simulink model "Robust_design_step_validation_2_2_4"  (R2024b)
settings: Solver=VariableStepAuto  StartTime=0.0  StopTime=20  FixedStep=0.001  RelTol=1e-3
undefined symbols (not defined in the file): degs2rpm, drv, gbox, index, K_vec, mld, mot, Nu, Nx, rads2rpm, rdp, rpm2rads, sens, Ts, u_bar_max
settings Model: Creator=Enrico  LastModifiedBy=Enrico 2
settings DataIOCC: ReturnWorkspaceOutputsName=out_black_box

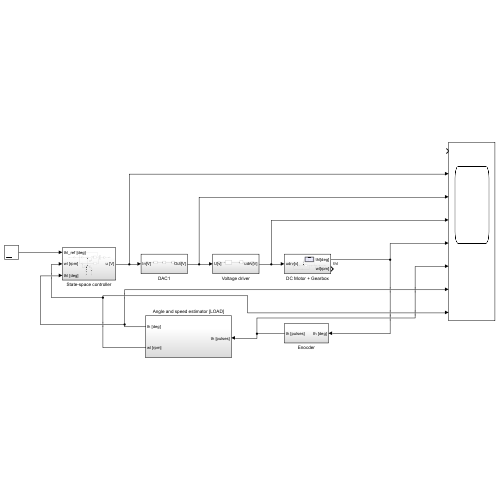
[thumbnail: Simulink's stored preview of the top-level diagram]
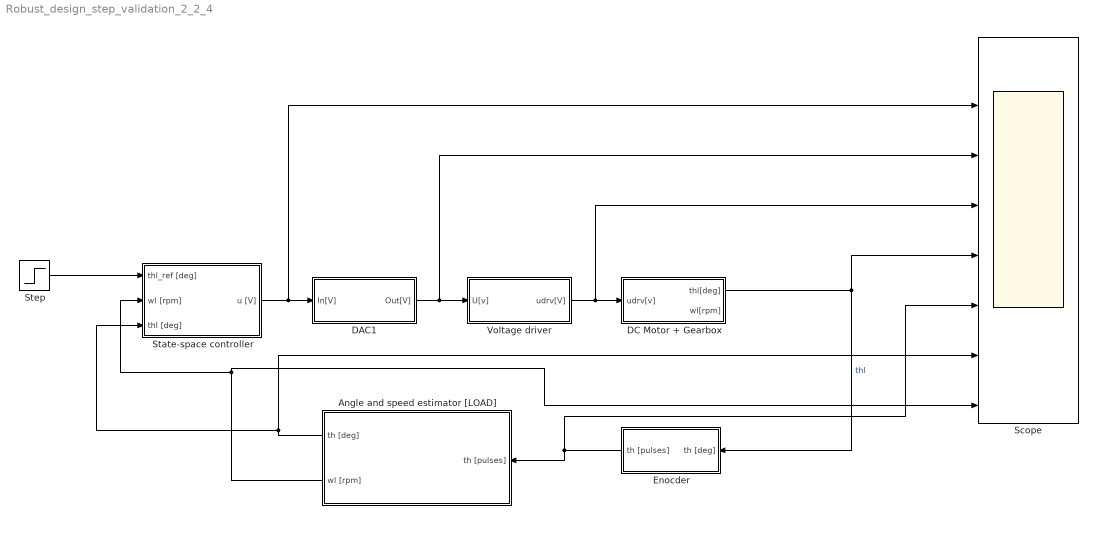
== system Robust_design_step_validation_2_2_4 ==
  Angle and speed estimator [LOAD] : Subsystem
  DAC1 : Subsystem
  DC Motor + Gearbox : Subsystem
  Enocder : Subsystem
  Scope : Scope  NumInputPorts=8
  State-space controller : Subsystem
  Step : Step  After=120  SampleTime=0
  Voltage driver : Subsystem
  wires:
  State-space controller/1(u [V]) -> DAC1/1(In[V]), Scope/2
  DAC1/1(Out[V]) -> Voltage driver/1(U[v]), Scope/3
  Step/1 -> State-space controller/1(thl_ref [deg])
  Enocder/1(th [pulses]) -> Scope/6, Angle and speed estimator [LOAD]/1(th [pulses])
  Voltage driver/1(udrv[V]) -> DC Motor + Gearbox/1(udrv[v]), Scope/4
  Angle and speed estimator [LOAD]/1(th [deg]) -> Scope/7, State-space controller/3(thl [deg])
  Angle and speed estimator [LOAD]/2(wl [rpm]) -> State-space controller/2(wl [rpm]), Scope/8
  DC Motor + Gearbox/1(thl[deg]) -> Enocder/1(th [deg]), Scope/5  "thl"

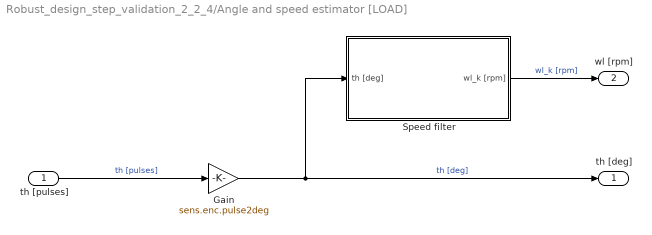
== system Robust_design_step_validation_2_2_4/Angle and speed estimator [LOAD] ==
  th [pulses] : Inport
  Gain : Gain  Gain=sens.enc.pulse2deg
  Speed filter : Subsystem
  th [deg] : Outport
  wl [rpm] : Outport  Port=2
  wires:
  Speed filter/1(wl_k [rpm]) -> wl [rpm]/1  "wl_k [rpm]"
  th [pulses]/1 -> Gain/1  "th [pulses]"
  Gain/1 -> Speed filter/1(th [deg]), th [deg]/1  "th [deg]"

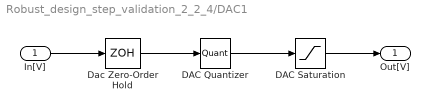
== system Robust_design_step_validation_2_2_4/DAC1 ==
  In[V] : Inport
  DAC Quantizer : Quantizer  QuantizationInterval=20/(2^16-1)
  DAC Saturation : Saturate  UpperLimit=10  LowerLimit=-10
  Dac Zero-Order Hold : ZeroOrderHold  SampleTime=Ts
  Out[V] : Outport
  wires:
  In[V]/1 -> Dac Zero-Order Hold/1
  DAC Saturation/1 -> Out[V]/1
  DAC Quantizer/1 -> DAC Saturation/1
  Dac Zero-Order Hold/1 -> DAC Quantizer/1

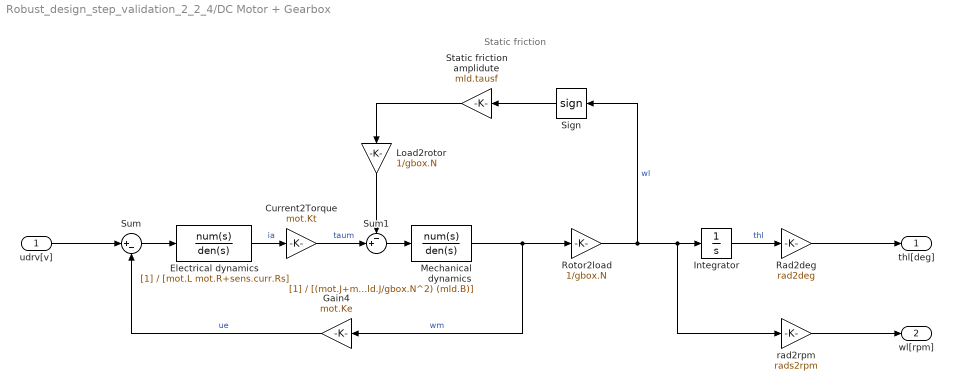
== system Robust_design_step_validation_2_2_4/DC Motor + Gearbox ==
  note: Static friction
  udrv[v] : Inport
  " Sign" : Signum  ZeroCross=off
  Current2Torque : Gain  Gain=mot.Kt
  Electrical dynamics : TransferFcn  Denominator=[mot.L mot.R+sens.curr.Rs]
  Gain4 : Gain  Gain=mot.Ke
  Integrator : Integrator
  Load2rotor : Gain  Gain=1/gbox.N
  Mechanical dynamics : TransferFcn  Denominator=[(mot.J+mld.J/gbox.N^2) (mld.B)]
  Rad2deg : Gain  Gain=rad2deg
  Rotor2load : Gain  Gain=1/gbox.N
  Static friction amplidute : Gain  Gain=mld.tausf
  Sum : Sum  Inputs=|+-
  Sum1 : Sum  Inputs=-+|
  rad2rpm : Gain  Gain=rads2rpm
  thl[deg] : Outport
  wl[rpm] : Outport  Port=2
  wires:
  udrv[v]/1 -> Sum/1
  Sum/1 -> Electrical dynamics/1
  Electrical dynamics/1 -> Current2Torque/1  "ia"
  Current2Torque/1 -> Sum1/2  "taum"
  Load2rotor/1 -> Sum1/1
  " Sign"/1 -> Static friction amplidute/1
  Static friction amplidute/1 -> Load2rotor/1
  Sum1/1 -> Mechanical dynamics/1
  Mechanical dynamics/1 -> Gain4/1, Rotor2load/1  "wm"
  Gain4/1 -> Sum/2  "ue"
  Rad2deg/1 -> thl[deg]/1
  rad2rpm/1 -> wl[rpm]/1
  Integrator/1 -> Rad2deg/1  "thl"
  Rotor2load/1 -> " Sign"/1, rad2rpm/1, Integrator/1  "wl"

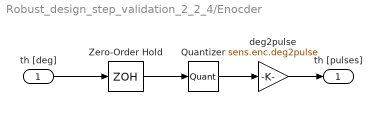
== system Robust_design_step_validation_2_2_4/Enocder ==
  th [deg] : Inport
  Quantizer : Quantizer  QuantizationInterval=sens.enc.pulse2deg
  Zero-Order Hold : ZeroOrderHold  SampleTime=Ts
  deg2pulse : Gain  Gain=sens.enc.deg2pulse
  th [pulses] : Outport
  wires:
  Quantizer/1 -> deg2pulse/1
  th [deg]/1 -> Zero-Order Hold/1
  Zero-Order Hold/1 -> Quantizer/1
  deg2pulse/1 -> th [pulses]/1

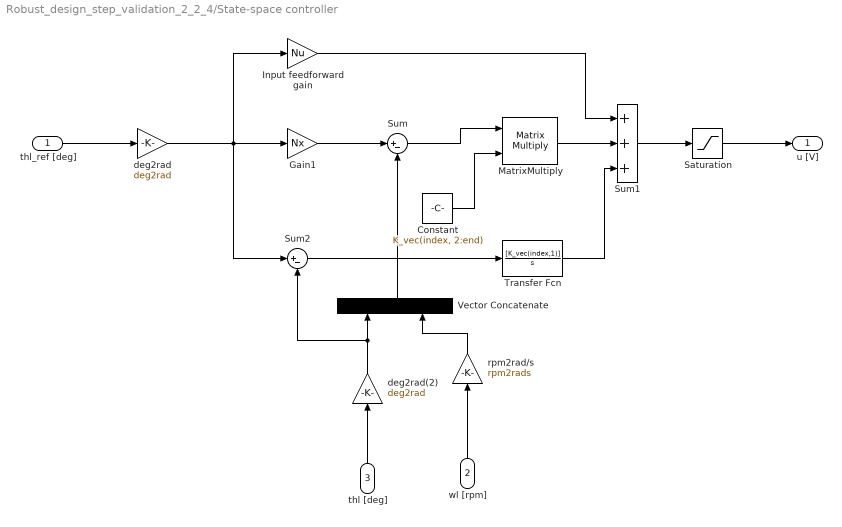
== system Robust_design_step_validation_2_2_4/State-space controller ==
  thl_ref [deg] : Inport
  wl [rpm] : Inport  Port=2
  thl [deg] : Inport  Port=3
  Constant : Constant  Value=K_vec(index, 2:end)
  Gain1 : Gain  Gain=Nx
  Input feedforward gain : Gain  Gain=Nu
  MatrixMultiply : Product  Multiplication=Matrix(*)
  Saturation : Saturate  UpperLimit=u_bar_max  LowerLimit=-u_bar_max
  Sum : Sum  Inputs=|+-
  Sum1 : Sum  Inputs=+++
  Sum2 : Sum  Inputs=|+-
  Transfer Fcn : TransferFcn  Numerator=[K_vec(index,1)]  Denominator=[1 0]
  Vector Concatenate : Concatenate
  deg2rad : Gain  Gain=deg2rad
  deg2rad(2) : Gain  Gain=deg2rad
  rpm2rad/s : Gain  Gain=rpm2rads
  u [V] : Outport
  wires:
  Gain1/1 -> Sum/1
  Sum1/1 -> Saturation/1
  deg2rad/1 -> Gain1/1, Sum2/1, Input feedforward gain/1
  thl_ref [deg]/1 -> deg2rad/1
  wl [rpm]/1 -> rpm2rad/s/1
  Input feedforward gain/1 -> Sum1/1
  Vector Concatenate/1 -> Sum/2
  Saturation/1 -> u [V]/1
  Sum/1 -> MatrixMultiply/1
  Constant/1 -> MatrixMultiply/2
  MatrixMultiply/1 -> Sum1/2
  Transfer Fcn/1 -> Sum1/3
  Sum2/1 -> Transfer Fcn/1
  thl [deg]/1 -> deg2rad(2)/1
  deg2rad(2)/1 -> Vector Concatenate/1, Sum2/2
  rpm2rad/s/1 -> Vector Concatenate/2

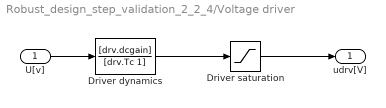
== system Robust_design_step_validation_2_2_4/Voltage driver ==
  U[v] : Inport
  Driver dynamics : TransferFcn  Numerator=[drv.dcgain]  Denominator=[drv.Tc 1]
  Driver saturation : Saturate  UpperLimit=12  LowerLimit=-12
  udrv[V] : Outport
  wires:
  U[v]/1 -> Driver dynamics/1
  Driver dynamics/1 -> Driver saturation/1
  Driver saturation/1 -> udrv[V]/1

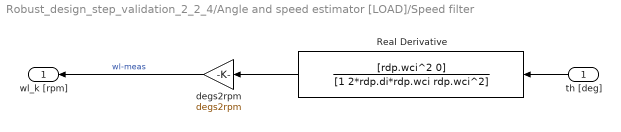
== system Robust_design_step_validation_2_2_4/Angle and speed estimator [LOAD]/Speed filter ==
  th [deg] : Inport
  Real Derivative : TransferFcn  Numerator=[rdp.wci^2 0]  Denominator=[1 2*rdp.di*rdp.wci rdp.wci^2]
  degs2rpm : Gain  Gain=degs2rpm
  wl_k [rpm] : Outport
  wires:
  th [deg]/1 -> Real Derivative/1
  degs2rpm/1 -> wl_k [rpm]/1  "wl-meas"
  Real Derivative/1 -> degs2rpm/1
